simulink library "DSCdq_Library"  (R2018a)
settings: Solver=VariableStepAuto  StartTime=0.0  StopTime=10.0  RelTol=1e-3
values from neighbouring files (symbols this model uses):
  Fcutout = 1000    [Application_Script.m]
  Fmin = 40    [Application_Script.m]
  Fn = 60    [Application_Script.m]    (also in ShortPulse_Script.m)
  Fsw = 6000    [Application_Script.m]
  Kp = 4    [Application_Script.m]
  Ti = L/R    (= 0.0530516476973)    [Application_Script.m]
  Ts = Ts_control / 60    (= 9.25925925926e-07)    [Application_Script.m]    (also in ShortPulse_Script.m)
  Ts_control = 1/(300*Fn)    (= 5.55555555556e-05)    [Application_Script.m]    (also in ShortPulse_Script.m)
  X = 0.5    [Application_Script.m]
  zeta = 2^-0.5    (= 0.707106781187)    [Application_Script.m]    (also in ShortPulse_Script.m)
undefined symbols (not defined in the file or in its folder): DiscIntNeverNeededParam, ESS, fn, Iap, PCC, Sn, tctrl, Uanp
libraries: $bdroot x54, powerlib_meascontrol x33, powerlib x3, cstblocks x2, simulink x2, peTransforms x2
(part 2 of 2)

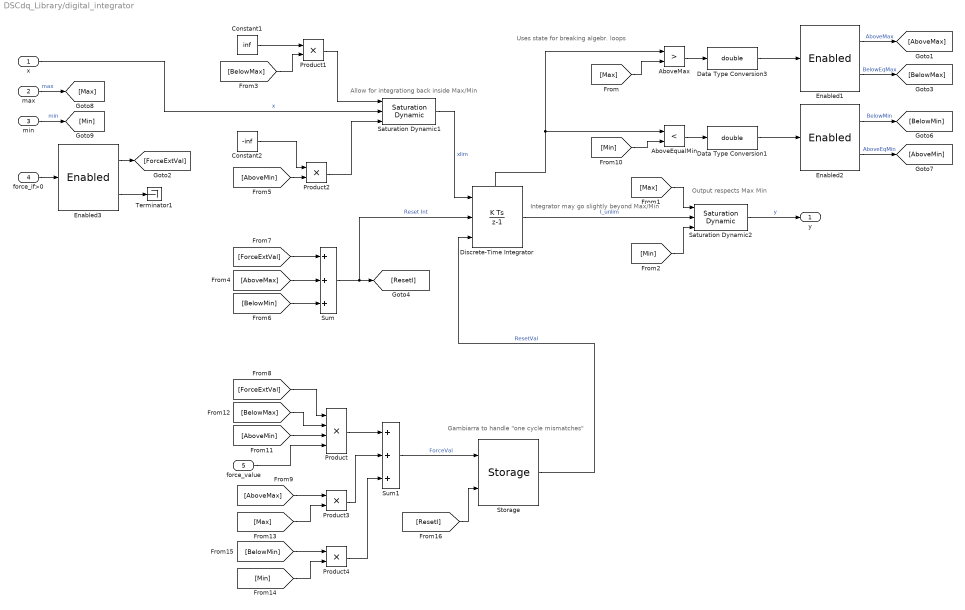
== system DSCdq_Library/digital_integrator ==
  note: Gambiarra to handle "one cycle mismatches"
  note: Integrator may go slightly beyond Max/Min
  note: Output respects Max Min
  note: Uses state for breaking algebr. loops
  note: Allow for integrationg back inside Max/Min
  x : Inport
  max : Inport  Port=2
  min : Inport  Port=3
  force_if>0 : Inport  Port=4
  force_value : Inport  Port=5
  AboveEqualMin : RelationalOperator  Operator=<  OutDataTypeStr=boolean  RndMeth=Simplest
  AboveMax : RelationalOperator  Operator=>  OutDataTypeStr=boolean  RndMeth=Simplest
  Constant1 : Constant  Value=inf
  Constant2 : Constant  Value=-inf
  Data Type Conversion1 : DataTypeConversion  OutDataTypeStr=double
  Data Type Conversion3 : DataTypeConversion  OutDataTypeStr=double
  Discrete-Time Integrator : DiscreteIntegrator  ExternalReset=level  InitialConditionSource=external  SampleTime=Ts  ShowStatePort=on  IgnoreLimit=on  ICPrevOutput=DiscIntNeverNeededParam  ICPrevScaledInput=DiscIntNeverNeededParam
  Enabled1 : $bdroot/Enabled
  Enabled2 : $bdroot/Enabled
  Enabled3 : $bdroot/Enabled
  Product : Product  Inputs=4
  Product{1..4} (4 alike) : Product
  Saturation Dynamic1 : simulink/Discontinuities/Saturation Dynamic  OutMin=[]  OutMax=[]  OutDataTypeStr=Inherit: Same as second input  OutDataType=fixdt(1, 16)  OutScaling=2^-10  DoSatur=off
  Saturation Dynamic2 : simulink/Discontinuities/Saturation Dynamic  OutMin=[]  OutMax=[]  OutDataTypeStr=Inherit: Same as second input  OutDataType=fixdt(1, 16)  OutScaling=2^-10  DoSatur=off
  Storage : $bdroot/Storage
  Sum : Sum  Inputs=+++
  Sum1 : Sum  Inputs=+++
  Terminator1 : Terminator
  y : Outport
  wires:
  x/1 -> Saturation Dynamic1/2  "x"
  Saturation Dynamic2/1 -> y/1  "y"
  max/1 -> [Max]  "max"
  min/1 -> [Min]  "min"
  force_value/1 -> Product/4
  Saturation Dynamic1/1 -> Discrete-Time Integrator/1  "xlim"
  [BelowMax] -> Product1/2
  Constant1/1 -> Product1/1
  Product1/1 -> Saturation Dynamic1/1
  [AboveMin] -> Product2/2
  Constant2/1 -> Product2/1
  Product2/1 -> Saturation Dynamic1/3
  Enabled1/1 -> [AboveMax]  "AboveMax"
  Enabled1/2 -> [BelowMax]  "BelowEqMax"
  Enabled2/2 -> [AboveMin]  "AboveEqMin"
  Enabled2/1 -> [BelowMin]  "BelowMin"
  [AboveMax] -> Sum/2
  [BelowMin] -> Sum/3
  force_if>0/1 -> Enabled3/1
  Enabled3/2 -> Terminator1/1
  [ForceExtVal] -> Product/1
  [AboveMax] -> Product3/1
  [Min] -> AboveEqualMin/2
  [AboveMin] -> Product/3
  [BelowMax] -> Product/2
  Product/1 -> Sum1/1
  [Max] -> Product3/2
  [BelowMin] -> Product4/1
  [Min] -> Product4/2
  Product4/1 -> Sum1/3
  Product3/1 -> Sum1/2
  Sum1/1 -> Storage/1  "ForceVal"
  Enabled3/1 -> [ForceExtVal]
  [Max] -> AboveMax/2
  Discrete-Time Integrator/1 -> Saturation Dynamic2/2  "I_unlim"
  [Max] -> Saturation Dynamic2/1
  [Min] -> Saturation Dynamic2/3
  AboveMax/1 -> Data Type Conversion3/1
  AboveEqualMin/1 -> Data Type Conversion1/1
  Data Type Conversion3/1 -> Enabled1/1
  Data Type Conversion1/1 -> Enabled2/1
  [ForceExtVal] -> Sum/1
  Discrete-Time Integrator/State -> AboveEqualMin/1, AboveMax/1
  Sum/1 -> Discrete-Time Integrator/2, [ResetI]  "Reset Int"
  [ResetI] -> Storage/2
  Storage/1 -> Discrete-Time Integrator/3  "ResetVal"

== system DSCdq_Library/dq_DSC ==
  x(k) : Inport
  n : Inport  Port=2
  CircBuffer_Delay_Ceil_Floor : $bdroot/CircBuffer_Delay_Ceil_Floor  Ts=Ts  nmax=nmax
  Constant : Constant
  Floor1 : Rounding  Operator=ceil
  Gain : Gain  Gain=0.5
  Multiply : Product
  Multiply1 : Product
  Sum1 : Sum  Inputs=+-
  Sum2 : Sum  Inputs=+-
  Sum3 : Sum
  Sum4 : Sum
  Sum5 : Sum
  y(k) : Outport
  wires:
  x(k)/1 -> Gain/1
  Sum3/1 -> Multiply/2  "y_ceil"
  Sum4/1 -> Multiply1/1  "y_floor"
  Constant/1 -> Sum1/1
  Sum2/1 -> Multiply1/2, Sum1/2
  Floor1/1 -> Sum2/1
  n/1 -> Sum2/2, Floor1/1, CircBuffer_Delay_Ceil_Floor/2
  Multiply1/1 -> Sum5/2
  Multiply/1 -> Sum5/1
  Sum1/1 -> Multiply/1
  Gain/1 -> Sum4/1, Sum3/1, CircBuffer_Delay_Ceil_Floor/1
  Sum5/1 -> y(k)/1  "y_w"
  CircBuffer_Delay_Ceil_Floor/1 -> Sum3/2
  CircBuffer_Delay_Ceil_Floor/2 -> Sum4/2

== system DSCdq_Library/idqref_gen_for_cnst_p ==
  vdq+ : Inport
  vdq- : Inport  Port=2
  idqref : Inport  Port=3
  MATLAB Function : MATLAB Function  TreatAsAtomicUnit=on  SystemSampleTime=Ts
  idqref- : Outport
  wires:
  MATLAB Function/1(idqref) -> idqref-/1
  vdq+/1 -> MATLAB Function/1(vdqp)
  vdq-/1 -> MATLAB Function/2(vdqn)
  idqref/1 -> MATLAB Function/3("idqref ")

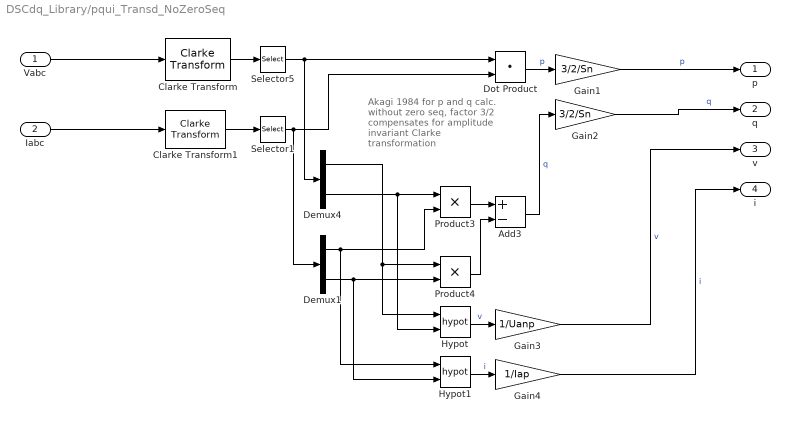
== system DSCdq_Library/pqui_Transd_NoZeroSeq ==
  note: Akagi 1984 for p and q
      | calc. without zero seq,
      | factor 3/2 compensates for
      | amplitude invariant
      | Clarke transformation
  Vabc : Inport
  Iabc : Inport  Port=2
  Add3 : Sum  Inputs=+-
  Clarke Transform : peTransforms/Clarke Transform  PowerInvariant=off
  Clarke Transform1 : peTransforms/Clarke Transform  PowerInvariant=off
  Demux1 : Demux  Outputs=2
  Demux4 : Demux  Outputs=2
  Dot Product : DotProduct  InputSameDT=on  OutDataTypeStr=Inherit: Inherit via internal rule
  Gain1 : Gain  Gain=3/2/Sn
  Gain2 : Gain  Gain=3/2/Sn
  Gain3 : Gain  Gain=1/Uanp
  Gain4 : Gain  Gain=1/Iap
  Hypot : Math  Operator=hypot  RndMeth=Zero  SaturateOnIntegerOverflow=on
  Hypot1 : Math  Operator=hypot  RndMeth=Zero  SaturateOnIntegerOverflow=on
  Product3 : Product
  Product4 : Product
  Selector1 : Selector  InputPortWidth=3  IndexOptions=Index vector (dialog)  Indices=[1 2]  OutputSizes=1
  Selector5 : Selector  InputPortWidth=3  IndexOptions=Index vector (dialog)  Indices=[1 2]  OutputSizes=1
  p : Outport
  q : Outport  Port=2
  v : Outport  Port=3
  i : Outport  Port=4
  wires:
  Clarke Transform1/1 -> Selector1/1
  Gain3/1 -> v/1  "v"
  Demux1/2 -> Hypot1/2, Product4/2
  Hypot1/1 -> Gain4/1  "i"
  Selector1/1 -> Demux1/1, Dot Product/2
  Selector5/1 -> Demux4/1, Dot Product/1
  Demux4/1 -> Hypot/1, Product4/1
  Hypot/1 -> Gain3/1  "v"
  Dot Product/1 -> Gain1/1  "p"
  Demux1/1 -> Hypot1/1, Product3/2
  Add3/1 -> Gain2/1  "q"
  Product4/1 -> Add3/2
  Demux4/2 -> Hypot/2, Product3/1
  Vabc/1 -> Clarke Transform/1
  Clarke Transform/1 -> Selector5/1
  Iabc/1 -> Clarke Transform1/1
  Product3/1 -> Add3/1
  Gain1/1 -> p/1  "p"
  Gain4/1 -> i/1  "i"
  Gain2/1 -> q/1  "q"

== matlab function DSCdq_Library/3waySelector/MATLAB Function ==
  data: In input; En0 output; Dis0 output; En1 output; Dis1 output; En2 output; Dis2 output
%%%%%%%%%%%%%%%%%%%%%%%%%%%%%%%%%%%%%%%%%%%%%%%%%%%%%%%%%%%%%%%%%%%%%%%%%%
% 3 way selector
%%%%%%%%%%%%%%%%%%%%%%%%%%%%%%%%%%%%%%%%%%%%%%%%%%%%%%%%%%%%%%%%%%%%%%%%%%\

%%%%%%%%%%%%%%%%%%%%%%%%%%%%%%%%%%%%%%%%%%%%%%%%%%%%%%%%%%%%%%%%%%%%%%%%%%\
% Prog/rev history
%   Mota - 2021-08-16: first release

function [En0,Dis0,En1,Dis1,En2,Dis2] = Enabled(In)

if In < 0.5
    En0 = 1;
    Dis0 = 0;
    
    En1 = 0;
    Dis1 = 1;
    
    En2 = 0;
    Dis2 = 1;
    
elseif In < 1.5
    En0 = 0;
    Dis0 = 1;
    
    En1 = 1;
    Dis1 = 0;
    
    En2 = 0;
    Dis2 = 1;
    
else
    En0 = 0;
    Dis0 = 1;
    
    En1 = 0;
    Dis1 = 1;
    
    En2 = 1;
    Dis2 = 0;
end

== matlab function DSCdq_Library/CircBuffer_Delay_Ceil_Floor/MATLAB Function ==
  data: x input; yc output; n input; yf output; nmax input
function [yc,    yf]  = CircBuff_Delay_CeilFloor(x, n, nmax)
%% %%%%%%%%%%%%%%%%%%%%%%%%%%%%%%%%%%%%%%%%%%%%%%%%%%%%%%%%%%%%%%%%%%%%%%%%
% Circular Buffer 
% By: Mota
% Revision history:
%       2021-07-16: first release
%
%%Interface  
%   Inputs
%       x : must be a vector pf two values
%       n : delay in samples (float, ideal delay is time was continuous)
%       nmax : max size of circular buffer, ONLY used in FIRST CYCLE
%
%   Output
%       yc = x(k - ceil(n))
%       yf = x(k - floor(n))
% 

persistent CB       % circular buffer, created with zeros in first cycle
persistent ins_p    % insertion pointer, integer, zero -> Nmax-1
persistent Nmax     % Buffer lenght, updated ONLY in FIRST CYCLE


%% Initialization of persistent variables
if isempty(Nmax)
    if nmax < 5     % Hardcoded minimum lenght of buffer (arbitrary)
        Nmax = 5;
    else 
        Nmax = round(nmax); % No limit for maximum lenght of buffer 
    end
    
    CB = zeros(Nmax, 2);    % circular buffer
                            % Nmax lines x 2 columns 
                            % Column 1: ceiling 
                            % Column 2: floor
    
    ins_p = 0;      % Insertion pointer initialization
    
end

%% %%%%%%%%%%%%%%%%%%%%%%%%%%%%%%%%%%%%%%%%%%%%%%%%%%%%%%%%%%%%%%%%%%%%%%
% Insertion of current values
%%%%%%%%%%%%%%%%%%%%%%%%%%%%%%%%%%%%%%%%%%%%%%%%%%%%%%%%%%%%%%%%%%%%%%%%%
CB(ins_p + 1, 1) = x(1);    
CB(ins_p + 1, 2) = x(2);

%% %%%%%%%%%%%%%%%%%%%%%%%%%%%%%%%%%%%%%%%%%%%%%%%%%%%%%%%%%%%%%%%%%%%%%%
% Retrieval pointer calculation
%   Be careful with confusion of indices
%       Matlab index for array:     1, 2,... Nmax
%       Insertion pointer values:   0, 1,... Nmax - 1
%%%%%%%%%%%%%%%%%%%%%%%%%%%%%%%%%%%%%%%%%%%%%%%%%%%%%%%%%%%%%%%%%%%%%%%%%
if n >= 1       
    if n <= Nmax - 1    % if 1 >= n >= Nmax - 1 
                        % n cannot be equal to Nmax, or else the retrieval
                        % pointers retreat back to the the insertion
                        % pointer.
                                
        p_r_c = mod(ins_p - ceil(n), Nmax); % ceiling retrieval pointer
        p_r_f = mod(ins_p - floor(n), Nmax); % floor retrieval pointer
    
    else
        % The maximum delay is Nmax - 1
        p_r_c = mod(ins_p - Nmax - 1, Nmax);
        p_r_f = mod(ins_p - Nmax - 1, Nmax);
    end
else
    % Minimul delay is zero
    p_r_c = ins_p;
    p_r_f = ins_p;
end
    
%% %%%%%%%%%%%%%%%%%%%%%%%%%%%%%%%%%%%%%%%%%%%%%%%%%%%%%%%%%%%%%%%%%%%%%%
% Temporary variables with retrieved values
%   CB indexes: 1, 2, ... Nmax
%%%%%%%%%%%%%%%%%%%%%%%%%%%%%%%%%%%%%%%%%%%%%%%%%%%%%%%%%%%%%%%%%%%%%%%%%
col1_c = CB(p_r_c + 1, 1); 
col1_f = CB(p_r_f + 1, 1);

col2_c = CB(p_r_c + 1, 2);
col2_f = CB(p_r_f + 1, 2);

%% %%%%%%%%%%%%%%%%%%%%%%%%%%%%%%%%%%%%%%%%%%%%%%%%%%%%%%%%%%%%%%%%%%%%%%
% Outputs vectors
%%%%%%%%%%%%%%%%%%%%%%%%%%%%%%%%%%%%%%%%%%%%%%%%%%%%%%%%%%%%%%%%%%%%%%%%%
yc = [col1_c; col2_c];
yf = [col1_f; col2_f];

%% %%%%%%%%%%%%%%%%%%%%%%%%%%%%%%%%%%%%%%%%%%%%%%%%%%%%%%%%%%%%%%%%%%%%%%
% Update Outputs vectors
%%%%%%%%%%%%%%%%%%%%%%%%%%%%%%%%%%%%%%%%%%%%%%%%%%%%%%%%%%%%%%%%%%%%%%%%%
ins_p = mod(ins_p + 1, Nmax);

== matlab function DSCdq_Library/idqref_gen_for_cnst_p/MATLAB Function ==
  data: vdqp input; idqref output; vdqn input; idqref input
function idqref = fcn(vdqp,vdqn,idqref)

% Calculation of the negative sequence references for zeroing the active 
% power second harmonic oscillations
% 
% Derived independently from, but later noticed that the same line of
% reasoning was adopted by Chaudhary 2012 "Negative Sequence Current
% Control in Wind Power Plants With VSC-HVDC Connection"

% In "expanded" matrix form
% | idn | = - | -vdp  +vqp |^{-1} * | -vdn  +vqn | * | idp | 
% | iqn | =   | +vqp  +vdp |        | -vdn  +vqn |   | idq |
% In matrix form
%  idqn   = -   vdqp^{-1}         *      vdqn      *   idqp

%The matrix that will be inverted
vp = zeros(2);
vp(1,1) = -vdqp(1);
vp(1,2) = vdqp(2);
vp(2,1) = vdqp(2);
vp(2,2) = vdqp(1);

%check is vp is invertible
if det(vp) == 0
    idqref(1,1) = 0;
    idqref(2,1) = 0;
else
    %The matrix that is not inverted
    vn = zeros(2);
    vn(1,1) = -vdqn(1);
    vn(1,2) = vdqn(2);
    vn(2,1) = vdqn(2);
    vn(2,2) = vdqn(1);

    % idqn = - vdqp^{-1} * vdqn * idqp
    idqref = -vp\vn*idqref;
end

== matlab function DSCdq_Library/Enabled/MATLAB Function ==
  data: En input; Enabled output; Disabled output
%%%%%%%%%%%%%%%%%%%%%%%%%%%%%%%%%%%%%%%%%%%%%%%%%%%%%%%%%%%%%%%%%%%%%%%%%%
% Enabled block
%%%%%%%%%%%%%%%%%%%%%%%%%%%%%%%%%%%%%%%%%%%%%%%%%%%%%%%%%%%%%%%%%%%%%%%%%%\

% Inputs
%   Enabled: if >0 enabled
% Output
%   Enabled: 1 if enabled, 0 if disabled
%   Disabled: 1 if disabled, 0 if enabled

%%%%%%%%%%%%%%%%%%%%%%%%%%%%%%%%%%%%%%%%%%%%%%%%%%%%%%%%%%%%%%%%%%%%%%%%%%\
% Prog/rev history
%   Mota - 2021-06-02: first release

function [Enabled,Disabled] = Enabled(En)

if En > 0
    Enabled = 1;
    Disabled = 0;
else
    Enabled = 0;
    Disabled = 1;
end

== matlab function DSCdq_Library/Storage/MATLAB Function ==
  data: x input; y output; store input
%%%%%%%%%%%%%%%%%%%%%%%%%%%%%%%%%%%%%%%%%%%%%%%%%%%%%%%%%%%%%%%%%%%%%%%%%%
% Storage block
%%%%%%%%%%%%%%%%%%%%%%%%%%%%%%%%%%%%%%%%%%%%%%%%%%%%%%%%%%%%%%%%%%%%%%%%%%\

% Inputs
%   Store: if > 0 store input
%   x = input
% Output
%   y = output

%%%%%%%%%%%%%%%%%%%%%%%%%%%%%%%%%%%%%%%%%%%%%%%%%%%%%%%%%%%%%%%%%%%%%%%%%%\
% Prog/rev history
%   Mota - 2021-06-02: first release

function y  = Store(x, store)

persistent dado

if isempty(dado)
    dado = 0;
end

if store <= 0
    y = dado;
    return
else
    y = x;
    dado = x;
end
